simulink model "headingSetpointCaclulation_th"  (R2018a)
settings: Solver=FixedStepDiscrete  StartTime=0.0  StopTime=1  FixedStep=0.1  RelTol=1e-3
undefined symbols (not defined in the file or in its folder): p, pos
libraries: headingSetpointCaclulation x1
settings Model: Creator=mitch  LastModifiedBy=mitch

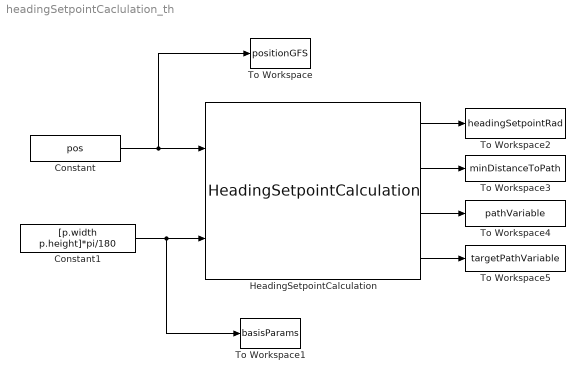
== system headingSetpointCaclulation_th ==
  Constant : Constant  Value=pos
  Constant1 : Constant  Value=[p.width p.height]*pi/180
  HeadingSetpointCalculation : headingSetpointCaclulation/HeadingSetpointCalculation  searchDistance=p.searchDistance  tol=p.projectionTolerance  meanElev=p.elev  leadLength=p.leadLength  initialPathVariable=p.initialPathVariable
  To Workspace : ToWorkspace  VariableName=positionGFS  SaveFormat=Timeseries  SampleTime=-1
  To Workspace1 : ToWorkspace  VariableName=basisParams  SaveFormat=Timeseries  SampleTime=-1
  To Workspace2 : ToWorkspace  VariableName=headingSetpointRad  SaveFormat=Timeseries  SampleTime=-1
  To Workspace3 : ToWorkspace  VariableName=minDistanceToPath  SaveFormat=Timeseries  SampleTime=-1
  To Workspace4 : ToWorkspace  VariableName=pathVariable  SaveFormat=Timeseries  SampleTime=-1
  To Workspace5 : ToWorkspace  VariableName=targetPathVariable  SaveFormat=Timeseries  SampleTime=-1
  wires:
  Constant/1 -> To Workspace/1, HeadingSetpointCalculation/1
  HeadingSetpointCalculation/2 -> To Workspace3/1
  HeadingSetpointCalculation/1 -> To Workspace2/1
  HeadingSetpointCalculation/3 -> To Workspace4/1
  HeadingSetpointCalculation/4 -> To Workspace5/1
  Constant1/1 -> To Workspace1/1, HeadingSetpointCalculation/2
